simulink model "RBD_linearizationattempt"  (R2022a)
settings: Solver=VariableStepAuto  StartTime=0.0  StopTime=10.0  RelTol=1e-3
model workspace (MAT data in the model file):
  op_trim1 = opcond.OperatingReport
  op_trim1.Outputs_(1) = opcond.OutputReport
  op_trim1.Outputs_(1).yspec_ = 0
  op_trim1.Outputs_(1).Block_ = 'RBD_linearizationattempt/Outport'
  op_trim1.Outputs_(1).PortWidth_ = 1
  op_trim1.Outputs_(1).PortNumber_ = NaN
  op_trim1.Outputs_(1).Known_ = 0
  op_trim1.Outputs_(1).Min_ = -Inf
  op_trim1.Outputs_(1).Max_ = Inf
  op_trim1.Outputs_(2) = opcond.OutputReport
  op_trim1.Outputs_(2).yspec_ = 0
  op_trim1.Outputs_(2).Block_ = 'RBD_linearizationattempt/Outport1'
  op_trim1.Outputs_(2).PortWidth_ = 1
  op_trim1.Outputs_(2).PortNumber_ = NaN
  op_trim1.Outputs_(2).Known_ = 0
  op_trim1.Outputs_(2).Min_ = -Inf
  op_trim1.Outputs_(2).Max_ = Inf
  op_trim1.Outputs_(3) = opcond.OutputReport
  op_trim1.Outputs_(3).yspec_ = 0
  op_trim1.Outputs_(3).Block_ = 'RBD_linearizationattempt/Outport2'
  op_trim1.Outputs_(3).PortWidth_ = 1
  op_trim1.Outputs_(3).PortNumber_ = NaN
  op_trim1.Outputs_(3).Known_ = 0
  op_trim1.Outputs_(3).Min_ = -Inf
  op_trim1.Outputs_(3).Max_ = Inf
  op_trim1.TerminationString_ = 'Operating point specifications were successfully met.'
  op_trim1.OptimizationOutput_.iterations = 2
  op_trim1.OptimizationOutput_.funcCount = 35
  op_trim1.OptimizationOutput_.lssteplength = 1
  op_trim1.OptimizationOutput_.stepsize = 3.50832904394e-12
  op_trim1.OptimizationOutput_.algorithm = 'active-set'
  op_trim1.OptimizationOutput_.firstorderopt = 0
  op_trim1.OptimizationOutput_.constrviolation = 1.16944301465e-09
  op_trim1.OptimizationOutput_.message = 'Local minimum found that satisfies the constraints.
    | 
    | Optimization completed because the objective function is non-decreasing in 
    | feasible directions, to within the value of the optimality tolerance,
    | and constraints are satisfied to within the  value of the constraint tolerance.
    | 
    | <stopping criteria details>
    | 
    | Optimization completed: The first-order optimality measure, 0.000000e+00, is less
    | than options.OptimalityTolerance = 1.000000e-06, and the maximum constraint violation,
    | 1.169443e-09,is less than options.ConstraintTolerance = 1.000000e-06.'
  op_trim1.OptimizationOutput_.bestfeasible.x = [0; 0; 0; 0; 0; 0; 0; 0; 0; 0; 0; 0; 0.0294299999965; 0; 0; 0]
  op_trim1.OptimizationOutput_.bestfeasible.fval = 0
  op_trim1.OptimizationOutput_.bestfeasible.constrviolation = 1.16944301465e-09
  op_trim1.OptimizationOutput_.bestfeasible.firstorderopt = 0
  op_trim1.OptimizationOutput_.progress = {'<font face="monospaced"; size=3><BR>', 'Optimizing to solve for all desired dx/dt=0, x(k+1)-x(k)=0, and y=ydes.<BR>', ' <BR>', '(Maximum Error)  Block<BR>', ' ---------------------------------------------------------<BR>', '(9.81000e+00) RBD_linearizationattempt/RBD/6DOF (Euler Angles)/ub,vb,wb<BR>', '(1.16944e-09) RBD_linearizationattempt/RBD/6DOF (Euler Angles)/ub,vb,wb<BR>', '(1.16944e-09) RBD_linearizationattempt/RBD/6DOF (Euler Angles)/ub,vb,wb<BR>', ' <BR>', 'Operating point specifications were successfully met.<BR>'}
  op_trim1.Model_ = 'RBD_linearizationattempt'
  op_trim1.States_(1) = opcond.StateReport
  op_trim1.States_(1).dx_ = [0; 0; 0]
  op_trim1.States_(1).Nx_ = 3
  op_trim1.States_(1).Block_ = 'RBD_linearizationattempt/RBD/6DOF (Euler Angles)/p,q,r '
  op_trim1.States_(1).x_ = [0; 0; 0]
  op_trim1.States_(1).SteadyState_ = [1; 1; 1]
  op_trim1.States_(1).dxMin_ = [-Inf; -Inf; -Inf]
  op_trim1.States_(1).dxMax_ = [Inf; Inf; Inf]
  op_trim1.States_(1).Known_ = [0; 0; 0]
  op_trim1.States_(1).Min_ = [-Inf; -Inf; -Inf]
  op_trim1.States_(1).Max_ = [Inf; Inf; Inf]
  op_trim1.States_(2) = opcond.StateReport
  op_trim1.States_(2).dx_ = [0; 0; 1.16944301465e-09]
  op_trim1.States_(2).Nx_ = 3
  op_trim1.States_(2).Block_ = 'RBD_linearizationattempt/RBD/6DOF (Euler Angles)/ub,vb,wb'
  op_trim1.States_(2).x_ = [0; 0; 0]
  op_trim1.States_(2).SteadyState_ = [1; 1; 1]
  op_trim1.States_(2).dxMin_ = [-Inf; -Inf; -Inf]
  op_trim1.States_(2).dxMax_ = [Inf; Inf; Inf]
  op_trim1.States_(2).Known_ = [0; 0; 0]
  op_trim1.States_(2).Min_ = [-Inf; -Inf; -Inf]
  op_trim1.States_(2).Max_ = [Inf; Inf; Inf]
  op_trim1.States_(3) = opcond.StateReport
  op_trim1.States_(3).dx_ = [0; 0; 0]
  op_trim1.States_(3).Nx_ = 3
  op_trim1.States_(3).Block_ = 'RBD_linearizationattempt/RBD/6DOF (Euler Angles)/xe,ye,ze'
  op_trim1.States_(3).x_ = [0; 0; 0]
  op_trim1.States_(3).SteadyState_ = [0; 0; 0]
  op_trim1.States_(3).dxMin_ = [-Inf; -Inf; -Inf]
  op_trim1.States_(3).dxMax_ = [Inf; Inf; Inf]
  op_trim1.States_(3).Known_ = [0; 0; 0]
  op_trim1.States_(3).Min_ = [-Inf; -Inf; -Inf]
  op_trim1.States_(3).Max_ = [Inf; Inf; Inf]
  op_trim1.States_(4) = opcond.StateReport
  op_trim1.States_(4).dx_ = [0; 0; 0]
  op_trim1.States_(4).Nx_ = 3
  op_trim1.States_(4).Block_ = 'RBD_linearizationattempt/RBD/6DOF (Euler Angles)/Calculate DCM &
    | Euler Angles/phi
    | theta
    | psi'
  op_trim1.States_(4).x_ = [0; 0; 0]
  op_trim1.States_(4).SteadyState_ = [1; 1; 1]
  op_trim1.States_(4).dxMin_ = [-Inf; -Inf; -Inf]
  op_trim1.States_(4).dxMax_ = [Inf; Inf; Inf]
  op_trim1.States_(4).Known_ = [0; 0; 0]
  op_trim1.States_(4).Min_ = [-Inf; -Inf; -Inf]
  op_trim1.States_(4).Max_ = [Inf; Inf; Inf]
  op_trim1.Inputs_(1) = opcond.InputReport
  op_trim1.Inputs_(1).Block_ = 'RBD_linearizationattempt/Thrust'
  op_trim1.Inputs_(1).PortWidth_ = 1
  op_trim1.Inputs_(1).PortDimensions_ = [1 1]
  op_trim1.Inputs_(1).u_ = 0.0294299999965
  op_trim1.Inputs_(1).Known_ = 0
  op_trim1.Inputs_(1).Min_ = -Inf
  op_trim1.Inputs_(1).Max_ = Inf
  op_trim1.Inputs_(2) = opcond.InputReport
  op_trim1.Inputs_(2).Block_ = 'RBD_linearizationattempt/tauX'
  op_trim1.Inputs_(2).PortWidth_ = 1
  op_trim1.Inputs_(2).PortDimensions_ = [1 1]
  op_trim1.Inputs_(2).Known_ = 0
  op_trim1.Inputs_(2).Min_ = -Inf
  op_trim1.Inputs_(2).Max_ = Inf
  op_trim1.Inputs_(3) = opcond.InputReport
  op_trim1.Inputs_(3).Block_ = 'RBD_linearizationattempt/tauY'
  op_trim1.Inputs_(3).PortWidth_ = 1
  op_trim1.Inputs_(3).PortDimensions_ = [1 1]
  op_trim1.Inputs_(3).Known_ = 0
  op_trim1.Inputs_(3).Min_ = -Inf
  op_trim1.Inputs_(3).Max_ = Inf
  op_trim1.Inputs_(4) = opcond.InputReport
  op_trim1.Inputs_(4).Block_ = 'RBD_linearizationattempt/tauZ'
  op_trim1.Inputs_(4).PortWidth_ = 1
  op_trim1.Inputs_(4).PortDimensions_ = [1 1]
  op_trim1.Inputs_(4).Known_ = 0
  op_trim1.Inputs_(4).Min_ = -Inf
  op_trim1.Inputs_(4).Max_ = Inf
values from neighbouring files (symbols this model uses):
  g = 9.81    [LQRCalcs.m]    (also in cf_firstOrderStateMdl.m; init_parameters.m; main.m; parameters_buildingSimulink.m)
  m = 0.003    [LQRCalcs.m]    (also in cf_firstOrderStateMdl.m; init_parameters.m = 4.34; main.m = 4.34; parameters_buildingSimulink.m = 4.34)
libraries: shared6dof x1
settings Model: Creator=Drew Lab Computer 1  LastModifiedBy=Drew Lab Computer 1
settings DataIOCC: ExternalInput=getinputstruct(op_trim1)  InitialState=getstatestruct(op_trim1)  LoadExternalInput=on  LoadInitialState=on

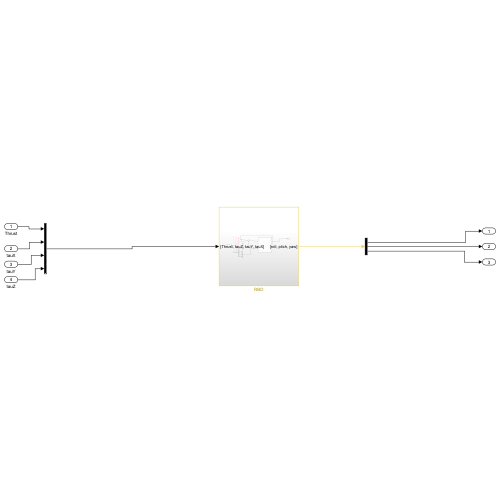
[thumbnail: Simulink's stored preview of the top-level diagram]
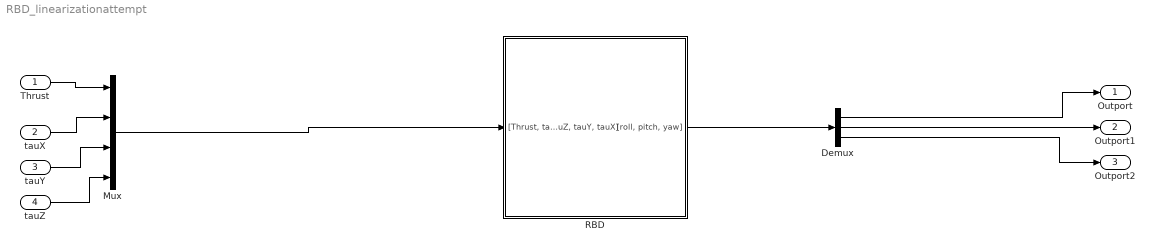
== system RBD_linearizationattempt ==
  Thrust : Inport
  tauX : Inport  Port=2
  tauY : Inport  Port=3
  tauZ : Inport  Port=4
  Demux : Demux  Outputs=3
  Mux : Mux
  RBD : Subsystem
  Outport : Outport
  Outport1 : Outport  Port=2
  Outport2 : Outport  Port=3
  wires:
  Thrust/1 -> Mux/1
  tauZ/1 -> Mux/4
  tauX/1 -> Mux/2
  tauY/1 -> Mux/3
  Mux/1 -> RBD/1("[Thrust, tauZ, tauY, tauX]")
  RBD/1("[roll, pitch, yaw]") -> Demux/1
  Demux/1 -> Outport/1
  Demux/2 -> Outport1/1
  Demux/3 -> Outport2/1

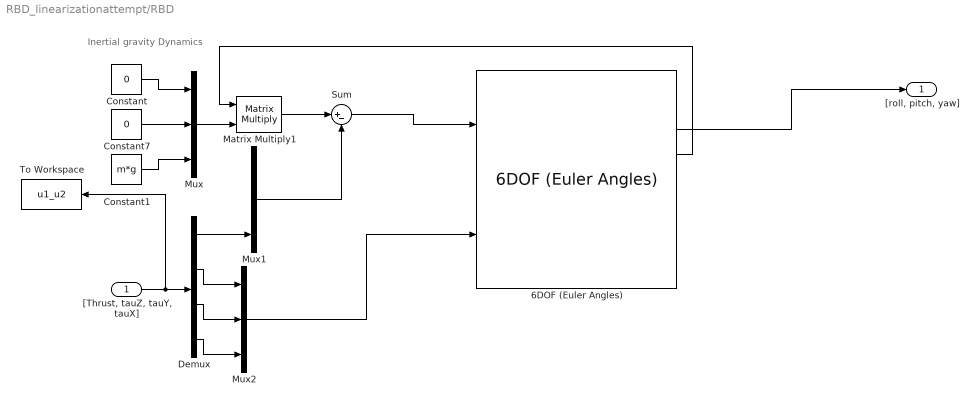
== system RBD_linearizationattempt/RBD ==
  note: Inertial gravity Dynamics
  "[Thrust, tauZ, tauY, tauX]" : Inport
  6DOF (Euler Angles) : shared6dof/6DOF (Euler Angles)  units=Metric (MKS)  mtype=Fixed  rep=Euler Angles  xme_0=X0  Vm_0=v0  eul_0=RPY_0  pm_0=pqr_0  mass_0=m  mass_e=0.5  mass_f=2.0  inertia=J  inertia_e=eye(3)  inertia_f=2*eye(3)  k_quat=1.0  vre_flag=on  abi_flag=on  aMode=0  xme_statename=''  Vm_statename=''  eul_statename=''  quat_statename=''  pm_statename=''  mass_statename=''
      settings: SourceProductBaseCode=AE,PW,DR,MT,VE
  Constant : Constant  Value=0
  Constant1 : Constant  Value=m*g
  Constant7 : Constant  Value=0
  Demux : Demux
  Matrix Multiply1 : Product  Multiplication=Matrix(*)
  Mux : Mux  Inputs=3
  Mux1 : Mux  Inputs=3
  Mux2 : Mux  Inputs=3
  Sum : Sum  Inputs=|+-
  To Workspace : ToWorkspace  VariableName=u1_u2  SaveFormat=Timeseries  SampleTime=-1
  "[roll, pitch, yaw]" : Outport
  wires:
  Sum/1 -> 6DOF (Euler Angles)/1
  Demux/3 -> Mux2/2
  Mux1/1 -> Sum/2
  Demux/4 -> Mux2/3
  Constant1/1 -> Mux/3
  Constant7/1 -> Mux/2
  Matrix Multiply1/1 -> Sum/1
  Demux/1 -> Mux1/3
  Constant/1 -> Mux/1
  Demux/2 -> Mux2/1
  6DOF (Euler Angles)/3 -> "[roll, pitch, yaw]"/1
  Mux/1 -> Matrix Multiply1/2
  "[Thrust, tauZ, tauY, tauX]"/1 -> Demux/1, To Workspace/1
  6DOF (Euler Angles)/4 -> Matrix Multiply1/1
  Mux2/1 -> 6DOF (Euler Angles)/2
